simulink model "model1"  (R2024b)
settings: Solver=VariableStepAuto  StartTime=0.0  StopTime=10.0  RelTol=1e-3
values from neighbouring files (symbols this model uses):
  A = -1    [run.m]
  Bw = [1,3]    [run.m]
  C = [1;2;3]    [run.m]
  Dw = [[1;2;3]*1+1,[ ... (first row only)    [run.m]
  L = inv(P)*Y    [run.m]
  Pival = eye(p)-C*pinv(C'*C)*C'    [run.m]
undefined symbols (not defined in the file or in its folder): Lmbda
libraries: simulink x1
settings Model: Creator=mehmetcanevi  LastModifiedBy=Mehmet

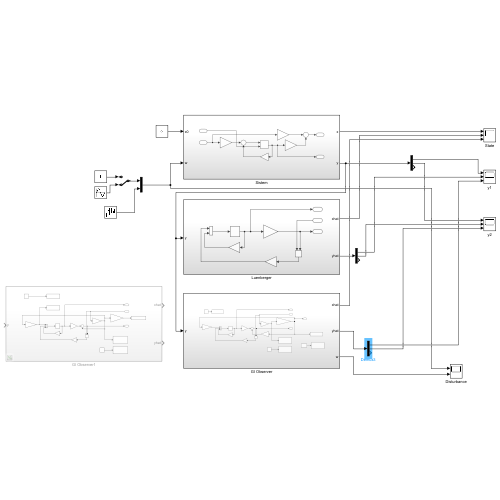
[thumbnail: Simulink's stored preview of the top-level diagram]
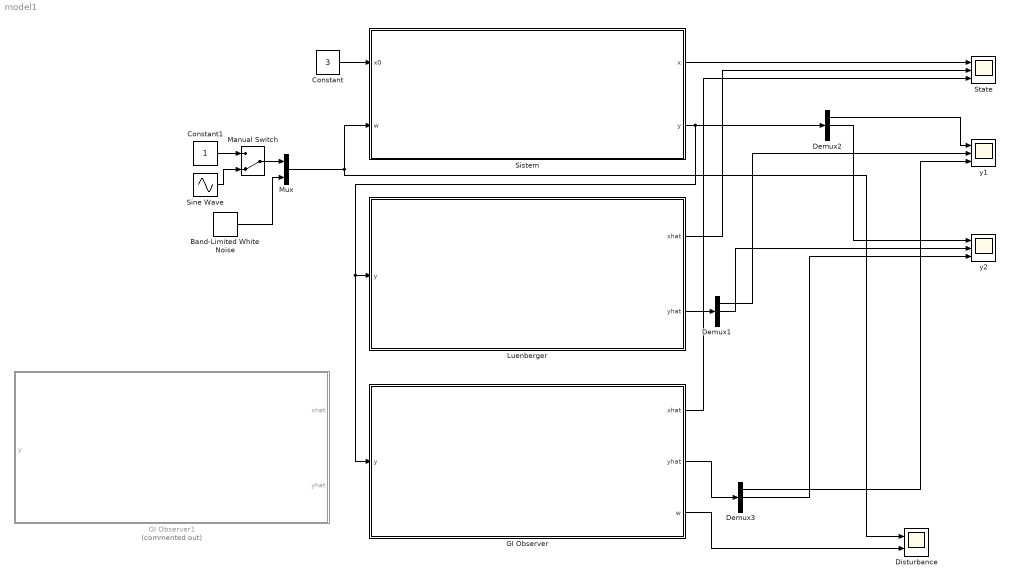
== system model1 ==
  Band-Limited White Noise : simulink/Sources/Band-Limited White Noise  Cov=1e-3  Ts=0.1  seed=[23341]
  Constant : Constant  Value=3
  Constant1 : Constant
  Demux1 : Demux  Outputs=3
  Demux2 : Demux  Outputs=3
  Demux3 : Demux  Outputs=3
  Disturbance : Scope  NumInputPorts=2
  GI Observer : Subsystem
  GI Observer1 : Subsystem  Commented=on
  Luenberger : Subsystem
  Manual Switch : ManualSwitch  CurrentSetting=0
  Mux : Mux  Inputs=2
  Sine Wave : Sin  SampleTime=0
  Sistem : Subsystem
  State : Scope  NumInputPorts=3
  y1 : Scope  NumInputPorts=3
  y2 : Scope  NumInputPorts=3
  wires:
  GI Observer/2(yhat) -> Demux3/1
  Constant/1 -> Sistem/1(x0)
  Sistem/1(x) -> State/1
  Luenberger/1(xhat) -> State/2
  GI Observer/1(xhat) -> State/3
  Demux2/1 -> y1/1
  Demux2/2 -> y2/1
  Luenberger/2(yhat) -> Demux1/1
  Demux1/1 -> y1/2
  Demux1/2 -> y2/2
  Demux3/1 -> y1/3
  Demux3/2 -> y2/3
  Mux/1 -> Disturbance/1, Sistem/2(w)
  GI Observer/3(w) -> Disturbance/2
  Sine Wave/1 -> Manual Switch/2
  Constant1/1 -> Manual Switch/1
  Sistem/2(y) -> GI Observer/1(y), Luenberger/1(y), Demux2/1
  Manual Switch/1 -> Mux/1
  Band-Limited White Noise/1 -> Mux/2

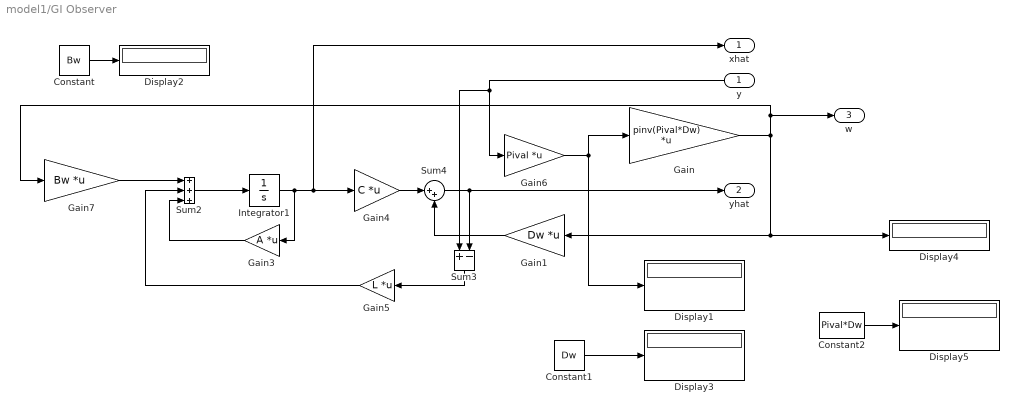
== system model1/GI Observer ==
  y : Inport
  Constant : Constant  Value=Bw
  Constant1 : Constant  Value=Dw
  Constant2 : Constant  Value=Pival*Dw
  Display{1..5} (5 alike) : Display
  Gain : Gain  Gain=pinv(Pival*Dw)  Multiplication=Matrix(K*u)
  Gain1 : Gain  Gain=Dw  Multiplication=Matrix(K*u)
  Gain3 : Gain  Gain=A  Multiplication=Matrix(K*u)
  Gain4 : Gain  Gain=C  Multiplication=Matrix(K*u)
  Gain5 : Gain  Gain=L  Multiplication=Matrix(K*u)
  Gain6 : Gain  Gain=Pival  Multiplication=Matrix(K*u)
  Gain7 : Gain  Gain=Bw  Multiplication=Matrix(K*u)
  Integrator1 : Integrator
  Sum2 : Sum  Inputs=+++
  Sum3 : Sum  Inputs=+-
  Sum4 : Sum  Inputs=|++
  xhat : Outport
  yhat : Outport  Port=2
  w : Outport  Port=3
  wires:
  Integrator1/1 -> xhat/1, Gain4/1, Gain3/1
  Sum2/1 -> Integrator1/1
  Gain6/1 -> Display1/1, Gain/1
  Gain7/1 -> Sum2/1
  Sum3/1 -> Gain5/1
  Gain3/1 -> Sum2/3
  y/1 -> Sum3/1, Gain6/1
  Gain5/1 -> Sum2/2
  Gain4/1 -> Sum4/1
  Sum4/1 -> Sum3/2, yhat/1
  Constant/1 -> Display2/1
  Constant1/1 -> Display3/1
  Gain/1 -> w/1, Gain7/1, Gain1/1, Display4/1
  Gain1/1 -> Sum4/2
  Constant2/1 -> Display5/1

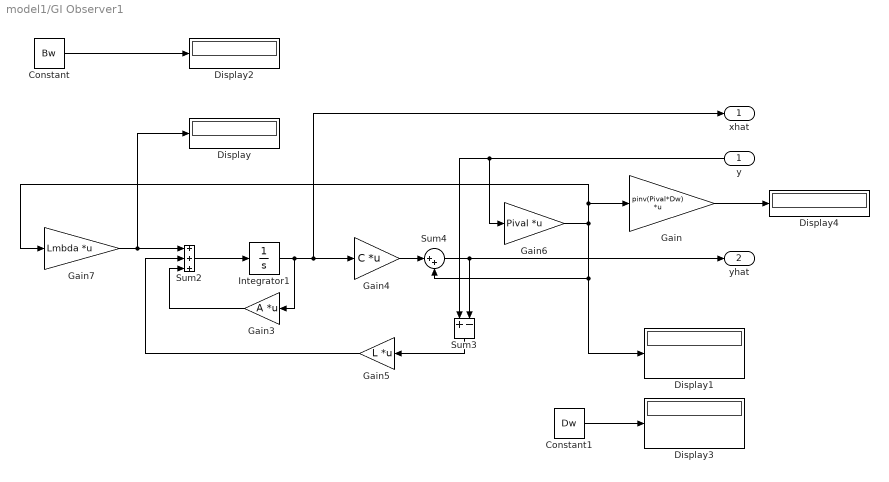
== system model1/GI Observer1 ==
  y : Inport
  Constant : Constant  Value=Bw
  Constant1 : Constant  Value=Dw
  Display{,1..4} (5 alike) : Display
  Gain : Gain  Gain=pinv(Pival*Dw)  Multiplication=Matrix(K*u)
  Gain3 : Gain  Gain=A  Multiplication=Matrix(K*u)
  Gain4 : Gain  Gain=C  Multiplication=Matrix(K*u)
  Gain5 : Gain  Gain=L  Multiplication=Matrix(K*u)
  Gain6 : Gain  Gain=Pival  Multiplication=Matrix(K*u)
  Gain7 : Gain  Gain=Lmbda  Multiplication=Matrix(K*u)
  Integrator1 : Integrator
  Sum2 : Sum  Inputs=+++
  Sum3 : Sum  Inputs=+-
  Sum4 : Sum  Inputs=|++
  xhat : Outport
  yhat : Outport  Port=2
  wires:
  Integrator1/1 -> xhat/1, Gain4/1, Gain3/1
  Sum2/1 -> Integrator1/1
  Gain6/1 -> Display1/1, Sum4/2, Gain/1, Gain7/1
  Gain7/1 -> Display/1, Sum2/1
  Sum3/1 -> Gain5/1
  Gain3/1 -> Sum2/3
  y/1 -> Sum3/1, Gain6/1
  Gain5/1 -> Sum2/2
  Gain4/1 -> Sum4/1
  Sum4/1 -> Sum3/2, yhat/1
  Constant/1 -> Display2/1
  Constant1/1 -> Display3/1
  Gain/1 -> Display4/1

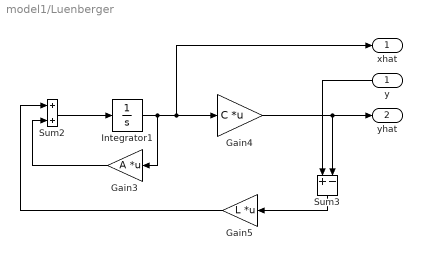
== system model1/Luenberger ==
  y : Inport
  Gain3 : Gain  Gain=A  Multiplication=Matrix(K*u)
  Gain4 : Gain  Gain=C  Multiplication=Matrix(K*u)
  Gain5 : Gain  Gain=L  Multiplication=Matrix(K*u)
  Integrator1 : Integrator
  Sum2 : Sum
  Sum3 : Sum  Inputs=+-
  xhat : Outport
  yhat : Outport  Port=2
  wires:
  Gain5/1 -> Sum2/1
  y/1 -> Sum3/1
  Gain3/1 -> Sum2/2
  Sum3/1 -> Gain5/1
  Gain4/1 -> Sum3/2, yhat/1
  Sum2/1 -> Integrator1/1
  Integrator1/1 -> Gain3/1, Gain4/1, xhat/1

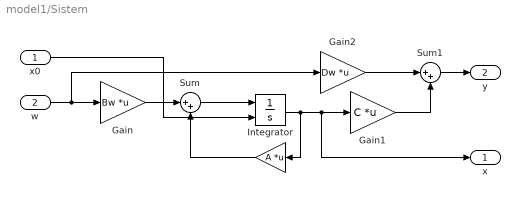
== system model1/Sistem ==
  x0 : Inport
  w : Inport  Port=2
  " " : Gain  Gain=A  Multiplication=Matrix(K*u)
  Gain : Gain  Gain=Bw  Multiplication=Matrix(K*u)
  Gain1 : Gain  Gain=C  Multiplication=Matrix(K*u)
  Gain2 : Gain  Gain=Dw  Multiplication=Matrix(K*u)
  Integrator : Integrator  InitialConditionSource=external
  Sum : Sum  Inputs=|++
  Sum1 : Sum  Inputs=|++
  x : Outport
  y : Outport  Port=2
  wires:
  Gain/1 -> Sum/1
  w/1 -> Gain2/1, Gain/1
  " "/1 -> Sum/2
  Gain2/1 -> Sum1/1
  Integrator/1 -> x/1, Gain1/1, " "/1
  Gain1/1 -> Sum1/2
  Sum1/1 -> y/1
  Sum/1 -> Integrator/1
  x0/1 -> Integrator/2
